simulink model "segway_sim"  (R2023a)
settings: Solver=VariableStepAuto  StartTime=0.0  StopTime=6.0  RelTol=1e-3
values from neighbouring files (symbols this model uses):
  Cinp = eye(2)    [segway_ini.m]
  Cout = [zeros(2,1), eye(2)]    [segway_ini.m]
  Cr2w = Cw2r^-1    [segway_ini.m]    (also in segway_planar_ini.m)
  Cw2r = [p.r/2     p.r/2;          p.r/p.b, -p.r/p.b]    [segway_ini.m]    (also in segway_planar_ini.m = [p.r])
  Ki = K(:,5:6)    [segway_ini.m]    (also in segway_planar_ini.m = K(:,4))
  Kx = K(:,1:4)    [segway_ini.m]    (also in segway_planar_ini.m = K(:,1:3))
  p = get_segway_params()    [segway_ini.m]    (also in segway_planar_ini.m)
libraries: cstblocks x3
settings Model: Creator=Michael Peter  LastModifiedBy=Michael Peter

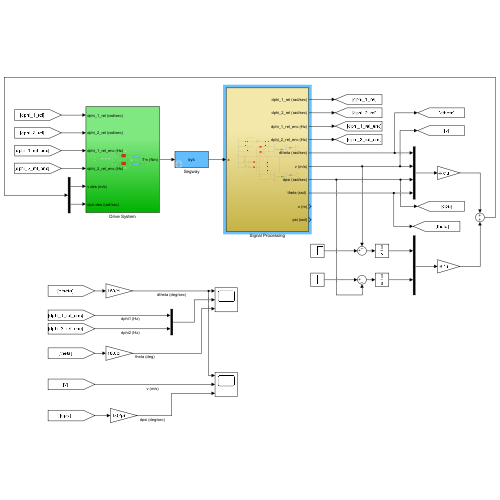
[thumbnail: Simulink's stored preview of the top-level diagram]
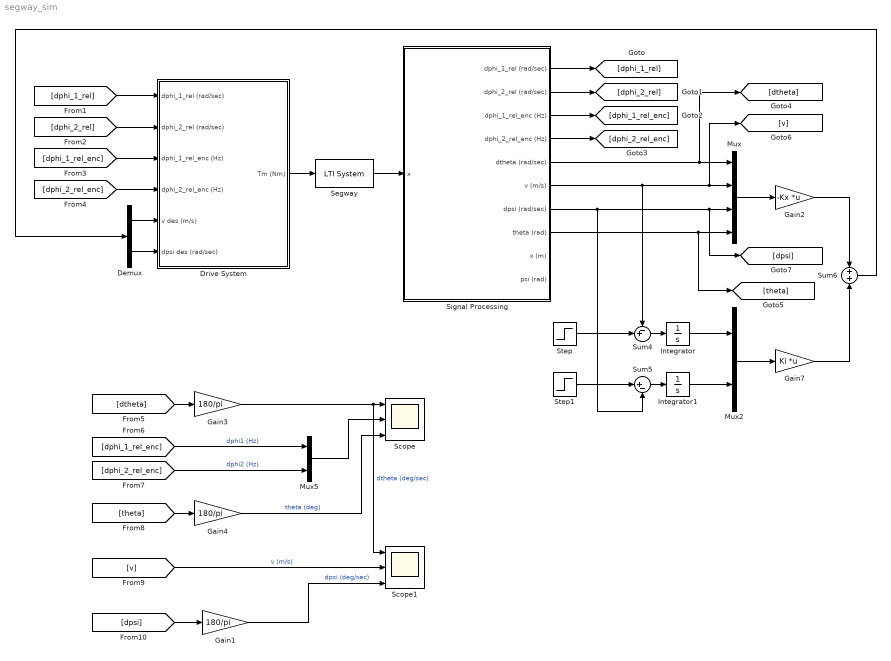
== system segway_sim ==
  Demux : Demux  Outputs=2
  Drive System : Subsystem
  Gain1 : Gain  Gain=180/pi
  Gain2 : Gain  Gain=-Kx  Multiplication=Matrix(K*u)
  Gain3 : Gain  Gain=180/pi
  Gain4 : Gain  Gain=180/pi
  Gain7 : Gain  Gain=Ki  Multiplication=Matrix(K*u)
  Integrator : Integrator
  Integrator1 : Integrator
  Mux : Mux
  Mux2 : Mux  Inputs=2
  Mux5 : Mux  Inputs=2
  Scope : Scope  NumInputPorts=3
  Scope1 : Scope  NumInputPorts=3
  Segway : cstblocks/LTI System  sys=sys  IC=x0
  Signal Processing : Subsystem
  Step : Step  Time=2  After=0.2  SampleTime=0
  Step1 : Step  Time=4  After=45*pi/180  SampleTime=0
  Sum4 : Sum  Inputs=-+|
  Sum5 : Sum  Inputs=|+-
  Sum6 : Sum  Inputs=+|+
  wires:
  Sum4/1 -> Integrator/1
  Sum5/1 -> Integrator1/1
  Mux2/1 -> Gain7/1
  [dtheta] -> Gain3/1
  [dphi_1_rel_enc] -> Mux5/1  "dphi1 (Hz)"
  [dphi_2_rel_enc] -> Mux5/2  "dphi2 (Hz)"
  Mux5/1 -> Scope/2
  [theta] -> Gain4/1
  Gain3/1 -> Scope1/1, Scope/1  "dtheta (deg/sec)"
  Gain4/1 -> Scope/3  "theta (deg)"
  Gain7/1 -> Sum6/2
  Integrator/1 -> Mux2/1
  Integrator1/1 -> Mux2/2
  Gain2/1 -> Sum6/1
  Signal Processing/8("theta (rad) ") -> [theta], Mux/4
  Signal Processing/6(v (m/s)) -> Sum4/1, [v], Mux/2
  Sum6/1 -> Demux/1
  Signal Processing/5(dtheta (rad/sec)) -> [dtheta], Mux/1
  Signal Processing/3(dphi_1_rel_enc (Hz)) -> [dphi_1_rel_enc]
  Signal Processing/1(dphi_1_rel (rad/sec)) -> [dphi_1_rel]
  Signal Processing/2(dphi_2_rel (rad/sec)) -> [dphi_2_rel]
  Signal Processing/4(dphi_2_rel_enc (Hz)) -> [dphi_2_rel_enc]
  [dphi_1_rel] -> Drive System/1(dphi_1_rel (rad/sec))
  [dphi_2_rel_enc] -> Drive System/4(dphi_2_rel_enc (Hz))
  [dphi_1_rel_enc] -> Drive System/3(dphi_1_rel_enc (Hz))
  [dphi_2_rel] -> Drive System/2(dphi_2_rel (rad/sec))
  Demux/1 -> Drive System/5(v des (m/s))
  Drive System/1(Tm (Nm)) -> Segway/1
  Demux/2 -> Drive System/6(dpsi des (rad/sec))
  Segway/1 -> Signal Processing/1(x)
  Signal Processing/7(dpsi (rad/sec)) -> Sum5/2, [dpsi], Mux/3
  Mux/1 -> Gain2/1
  Step/1 -> Sum4/2
  Step1/1 -> Sum5/1
  [dpsi] -> Gain1/1
  [v] -> Scope1/2  "v (m/s)"
  Gain1/1 -> Scope1/3  "dpsi (deg/sec)"

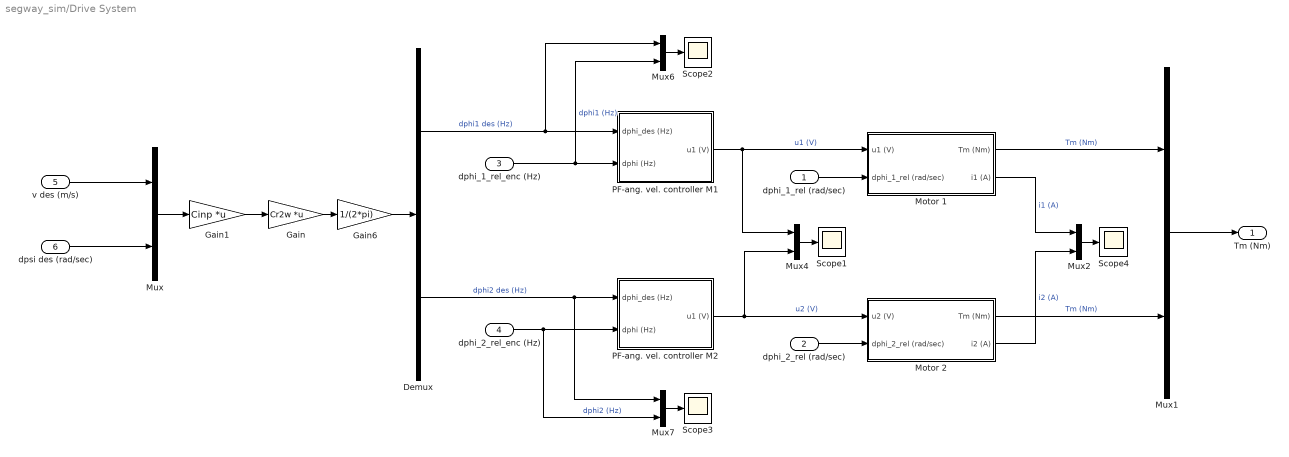
== system segway_sim/Drive System ==
  dphi_1_rel (rad/sec) : Inport
  dphi_2_rel (rad/sec) : Inport  Port=2
  dphi_1_rel_enc (Hz) : Inport  Port=3
  dphi_2_rel_enc (Hz) : Inport  Port=4
  v des (m/s) : Inport  Port=5
  dpsi des (rad/sec) : Inport  Port=6
  Demux : Demux  Outputs=2
  Gain : Gain  Gain=Cr2w  Multiplication=Matrix(K*u)
  Gain1 : Gain  Gain=Cinp  Multiplication=Matrix(K*u)
  Gain6 : Gain  Gain=1/(2*pi)
  Motor 1 : Subsystem
  Motor 2 : Subsystem
  Mux{,1..2,4,6..7} (6 alike) : Mux  Inputs=2
  PF-ang. vel. controller M1 : Subsystem
  PF-ang. vel. controller M2 : Subsystem
  Scope{1..4} (4 alike) : Scope
  Tm (Nm) : Outport
  wires:
  dphi_1_rel_enc (Hz)/1 -> PF-ang. vel. controller M1/2(dphi (Hz)), Mux6/2  "dphi1 (Hz)"
  dphi_1_rel (rad/sec)/1 -> Motor 1/2(dphi_1_rel (rad/sec))
  Motor 2/2(i2 (A)) -> Mux2/2  "i2 (A)"
  Mux4/1 -> Scope1/1
  Demux/1 -> PF-ang. vel. controller M1/1(dphi_des (Hz)), Mux6/1  "dphi1 des (Hz)"
  Demux/2 -> PF-ang. vel. controller M2/1(dphi_des (Hz)), Mux7/1  "dphi2 des (Hz)"
  Mux7/1 -> Scope3/1
  PF-ang. vel. controller M1/1(u1 (V)) -> Mux4/1, Motor 1/1(u1 (V))  "u1 (V)"
  Motor 1/1(Tm (Nm)) -> Mux1/1  "Tm (Nm)"
  dphi_2_rel_enc (Hz)/1 -> PF-ang. vel. controller M2/2(dphi (Hz)), Mux7/2  "dphi2 (Hz)"
  PF-ang. vel. controller M2/1(u1 (V)) -> Mux4/2, Motor 2/1(u2 (V))  "u2 (V)"
  Mux6/1 -> Scope2/1
  Motor 2/1(Tm (Nm)) -> Mux1/2  "Tm (Nm)"
  Mux1/1 -> Tm (Nm)/1
  dphi_2_rel (rad/sec)/1 -> Motor 2/2(dphi_2_rel (rad/sec))
  Motor 1/2(i1 (A)) -> Mux2/1  "i1 (A)"
  Mux2/1 -> Scope4/1
  dpsi des (rad/sec)/1 -> Mux/2
  v des (m/s)/1 -> Mux/1
  Mux/1 -> Gain1/1
  Gain6/1 -> Demux/1
  Gain/1 -> Gain6/1
  Gain1/1 -> Gain/1

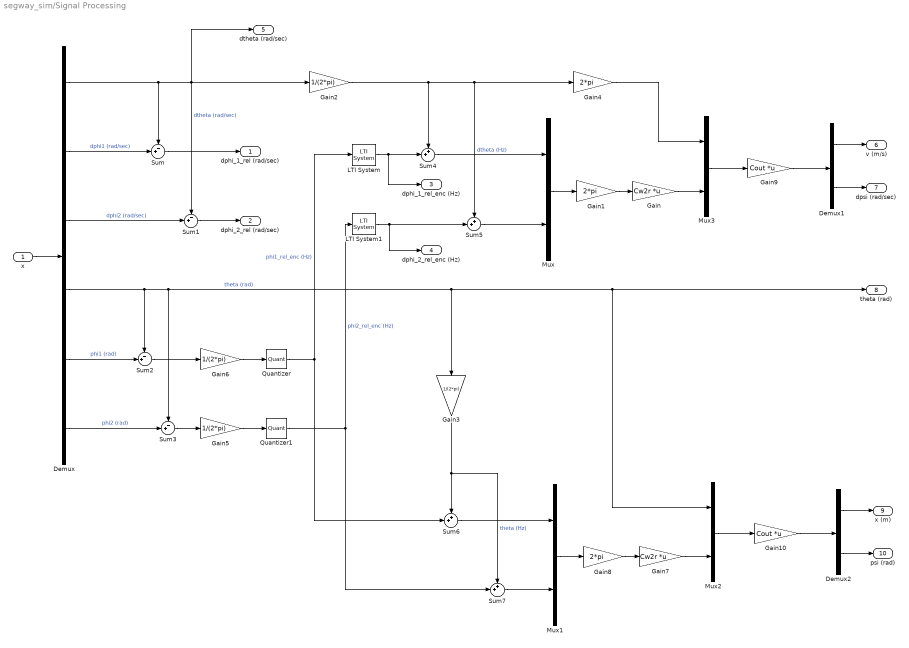
== system segway_sim/Signal Processing ==
  x : Inport
  Demux : Demux  Outputs=6
  Demux1 : Demux  Outputs=2
  Demux2 : Demux  Outputs=2
  Gain : Gain  Gain=Cw2r  Multiplication=Matrix(K*u)
  Gain1 : Gain  Gain=2*pi
  Gain10 : Gain  Gain=Cout  Multiplication=Matrix(K*u)
  Gain{2..3,5..6} (4 alike) : Gain  Gain=1/(2*pi)
  Gain4 : Gain  Gain=2*pi
  Gain7 : Gain  Gain=Cw2r  Multiplication=Matrix(K*u)
  Gain8 : Gain  Gain=2*pi
  Gain9 : Gain  Gain=Cout  Multiplication=Matrix(K*u)
  LTI System : cstblocks/LTI System  sys=Gfd  IC=[]
  LTI System1 : cstblocks/LTI System  sys=Gfd  IC=[]
  Mux{,1..3} (4 alike) : Mux  Inputs=2
  Quantizer : Quantizer  QuantizationInterval=1/p.CPR
  Quantizer1 : Quantizer  QuantizationInterval=1/p.CPR
  Sum{,1..3} (4 alike) : Sum  Inputs=-+|
  Sum{4..7} (4 alike) : Sum  Inputs=++|
  dphi_1_rel (rad/sec) : Outport
  dphi_2_rel (rad/sec) : Outport  Port=2
  dphi_1_rel_enc (Hz) : Outport  Port=3
  dphi_2_rel_enc (Hz) : Outport  Port=4
  dtheta (rad/sec) : Outport  Port=5
  v (m/s) : Outport  Port=6
  dpsi (rad/sec) : Outport  Port=7
  "theta (rad) " : Outport  Port=8
  x (m) : Outport  Port=9
  psi (rad) : Outport  Port=10
  wires:
  Demux/2 -> Sum/2  "dphi1 (rad/sec)"
  Demux/1 -> dtheta (rad/sec)/1, Sum1/1, Gain2/1, Sum/1  "dtheta (rad/sec)"
  Demux/3 -> Sum1/2  "dphi2 (rad/sec)"
  Sum/1 -> dphi_1_rel (rad/sec)/1
  Sum1/1 -> dphi_2_rel (rad/sec)/1
  Demux/6 -> Sum3/2  "phi2 (rad)"
  Demux/5 -> Sum2/2  "phi1 (rad)"
  Sum2/1 -> Gain6/1
  Sum3/1 -> Gain5/1
  Gain6/1 -> Quantizer/1
  Gain5/1 -> Quantizer1/1
  LTI System/1 -> dphi_1_rel_enc (Hz)/1, Sum4/2
  LTI System1/1 -> dphi_2_rel_enc (Hz)/1, Sum5/2
  x/1 -> Demux/1
  Mux/1 -> Gain1/1
  Sum4/1 -> Mux/1
  Sum5/1 -> Mux/2
  Gain2/1 -> Sum4/1, Gain4/1, Sum5/1  "dtheta (Hz)"
  Gain1/1 -> Gain/1
  Quantizer/1 -> Sum6/2, LTI System/1  "phi1_rel_enc (Hz)"
  Quantizer1/1 -> Sum7/2, LTI System1/1  "phi2_rel_enc (Hz)"
  Sum6/1 -> Mux1/1
  Sum7/1 -> Mux1/2
  Gain3/1 -> Sum7/1, Sum6/1  "theta (Hz)"
  Gain8/1 -> Gain7/1
  Mux1/1 -> Gain8/1
  Gain9/1 -> Demux1/1
  Demux1/2 -> dpsi (rad/sec)/1
  Demux1/1 -> v (m/s)/1
  Gain/1 -> Mux3/2
  Mux3/1 -> Gain9/1
  Demux2/1 -> x (m)/1
  Mux2/1 -> Gain10/1
  Gain10/1 -> Demux2/1
  Demux/4 -> Mux2/1, "theta (rad) "/1, Gain3/1, Sum3/1, Sum2/1  "theta (rad)"
  Gain7/1 -> Mux2/2
  Demux2/2 -> psi (rad)/1
  Gain4/1 -> Mux3/1

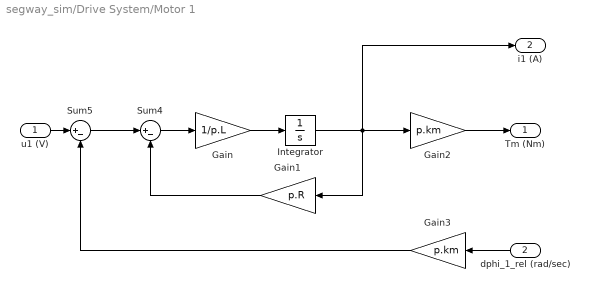
== system segway_sim/Drive System/Motor 1 ==
  u1 (V) : Inport
  dphi_1_rel (rad/sec) : Inport  Port=2
  Gain : Gain  Gain=1/p.L
  Gain1 : Gain  Gain=p.R
  Gain2 : Gain  Gain=p.km
  Gain3 : Gain  Gain=p.km
  Integrator : Integrator
  Sum4 : Sum  Inputs=|+-
  Sum5 : Sum  Inputs=|+-
  Tm (Nm) : Outport
  i1 (A) : Outport  Port=2
  wires:
  Integrator/1 -> Gain1/1, i1 (A)/1, Gain2/1
  Gain1/1 -> Sum4/2
  Gain3/1 -> Sum5/2
  u1 (V)/1 -> Sum5/1
  Sum5/1 -> Sum4/1
  Sum4/1 -> Gain/1
  Gain/1 -> Integrator/1
  dphi_1_rel (rad/sec)/1 -> Gain3/1
  Gain2/1 -> Tm (Nm)/1

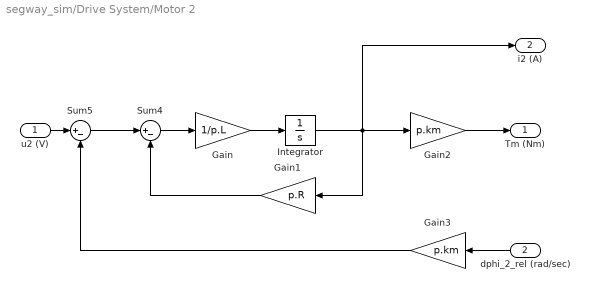
== system segway_sim/Drive System/Motor 2 ==
  u2 (V) : Inport
  dphi_2_rel (rad/sec) : Inport  Port=2
  Gain : Gain  Gain=1/p.L
  Gain1 : Gain  Gain=p.R
  Gain2 : Gain  Gain=p.km
  Gain3 : Gain  Gain=p.km
  Integrator : Integrator
  Sum4 : Sum  Inputs=|+-
  Sum5 : Sum  Inputs=|+-
  Tm (Nm) : Outport
  i2 (A) : Outport  Port=2
  wires:
  Gain2/1 -> Tm (Nm)/1
  dphi_2_rel (rad/sec)/1 -> Gain3/1
  Gain/1 -> Integrator/1
  Sum4/1 -> Gain/1
  Sum5/1 -> Sum4/1
  u2 (V)/1 -> Sum5/1
  Gain3/1 -> Sum5/2
  Gain1/1 -> Sum4/2
  Integrator/1 -> Gain2/1, i2 (A)/1, Gain1/1

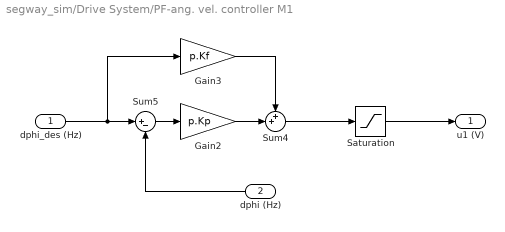
== system segway_sim/Drive System/PF-ang. vel. controller M1 ==
  dphi_des (Hz) : Inport
  dphi (Hz) : Inport  Port=2
  Gain2 : Gain  Gain=p.Kp
  Gain3 : Gain  Gain=p.Kf
  Saturation : Saturate  UpperLimit=p.u_max  LowerLimit=p.u_min
  Sum4 : Sum  Inputs=++|
  Sum5 : Sum  Inputs=|+-
  u1 (V) : Outport
  wires:
  Sum5/1 -> Gain2/1
  dphi_des (Hz)/1 -> Gain3/1, Sum5/1
  dphi (Hz)/1 -> Sum5/2
  Gain3/1 -> Sum4/1
  Gain2/1 -> Sum4/2
  Sum4/1 -> Saturation/1
  Saturation/1 -> u1 (V)/1

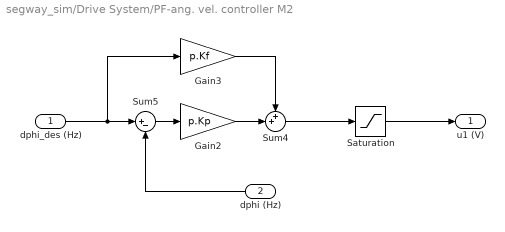
== system segway_sim/Drive System/PF-ang. vel. controller M2 ==
  dphi_des (Hz) : Inport
  dphi (Hz) : Inport  Port=2
  Gain2 : Gain  Gain=p.Kp
  Gain3 : Gain  Gain=p.Kf
  Saturation : Saturate  UpperLimit=p.u_max  LowerLimit=p.u_min
  Sum4 : Sum  Inputs=++|
  Sum5 : Sum  Inputs=|+-
  u1 (V) : Outport
  wires:
  Sum5/1 -> Gain2/1
  dphi_des (Hz)/1 -> Gain3/1, Sum5/1
  dphi (Hz)/1 -> Sum5/2
  Gain3/1 -> Sum4/1
  Gain2/1 -> Sum4/2
  Sum4/1 -> Saturation/1
  Saturation/1 -> u1 (V)/1
